simulink model "pid_handle_statico"  (R2018b)
settings: Solver=VariableStepAuto  StartTime=0.0  StopTime=10  RelTol=1e-3
values from neighbouring files (symbols this model uses):
  cond_init = [0, 150/180*pi, pi/3, -pi/2, -3*pi/4,-150/180*pi]'    [init.m]
  Legge = [Kp,Kd]    [LAUNCH_COMP_TORQUE_TRAJ.m]    (also in LAUNCH_PD.m = [Kp Kd]; LAUNCH_PD_TRAJ.m)
  param = param'    [init.m]
  q_position_f = [45/180*pi, 30*pi/180, 60*pi/180 ,90*pi/180, -45*pi/180, 330*pi/180]'    [init.m]
settings Model: Creator=Utente  LastModifiedBy=Utente

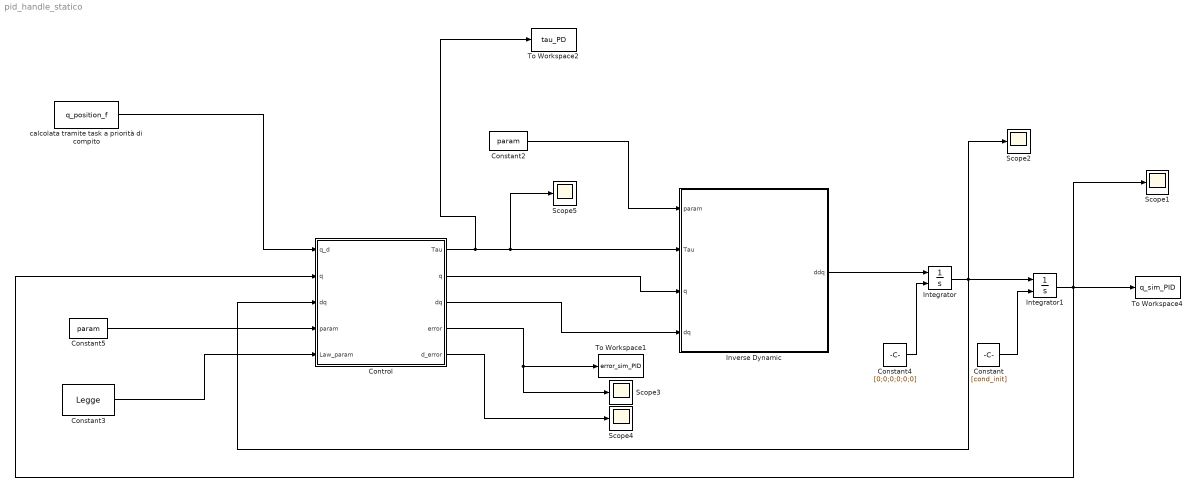
== system pid_handle_statico ==
  Constant : Constant  Value=[cond_init]
  Constant2 : Constant  Value=param
  Constant3 : Constant  Value=Legge
  Constant4 : Constant  Value=[0;0;0;0;0;0]
  Constant5 : Constant  Value=param
  Control : MATLAB Function  TreatAsAtomicUnit=on
  Integrator : Integrator  InitialConditionSource=external  InitialCondition=[0;0;0;0;0;0]
  Integrator1 : Integrator  InitialConditionSource=external
  Inverse Dynamic : MATLAB Function  TreatAsAtomicUnit=on
  Scope{1..5} (5 alike) : Scope
  To Workspace1 : ToWorkspace  VariableName=error_sim_PID  SaveFormat=Structure With Time  SampleTime=-1
      settings: Save2DSignal=2-D array (concatenate along first dimension)
  To Workspace2 : ToWorkspace  VariableName=tau_PD  SaveFormat=Structure With Time  SampleTime=-1
      settings: Save2DSignal=2-D array (concatenate along first dimension)
  To Workspace4 : ToWorkspace  VariableName=q_sim_PID  SaveFormat=Structure With Time  SampleTime=-1
      settings: Save2DSignal=2-D array (concatenate along first dimension)
  calcolata tramite task a priorità di compito : Constant  Value=q_position_f
  wires:
  Constant2/1 -> Inverse Dynamic/1(param)
  Constant3/1 -> Control/5(Law_param)
  Control/1(Tau) -> To Workspace2/1, Scope5/1, Inverse Dynamic/2(Tau)
  Control/2(q) -> Inverse Dynamic/3(q)
  Integrator/1 -> Control/3("dq "), Integrator1/1, Scope2/1
  Inverse Dynamic/1(ddq) -> Integrator/1
  Constant/1 -> Integrator1/2
  Integrator1/1 -> Control/2("q "), To Workspace4/1, Scope1/1
  Constant4/1 -> Integrator/2
  Control/3(dq) -> Inverse Dynamic/4(dq)
  calcolata tramite task a priorità di compito/1 -> Control/1(q_d)
  Constant5/1 -> Control/4(param)
  Control/4(error) -> To Workspace1/1, Scope3/1
  Control/5(d_error) -> Scope4/1

== matlab function pid_handle_statico/Control ==
  data: q_d input; q input; dq input; Tau output; param input; Law_param input; q output; dq output; error output; d_error output
function [Tau,q,dq, error, d_error] = ControlLaw(q_d, q, dq,  param, Law_param)

Kp = Law_param(1)*eye(size(q,1));
Kd = Law_param(2)*eye(size(dq,1));

[~,~,G] = Dinamica_new(param,q,dq);

error = q_d - q;
d_error = - dq;

Tau = Kp*error + G - Kd*dq;

end

== matlab function pid_handle_statico/Inverse Dynamic ==
  data: param input; Tau input; ddq output; q input; dq input
function ddq = inverseD(param,Tau,q,dq)

    [B,C,G] = Dinamica(param,q,dq);
    tot = Tau - C*dq - G;
    
    ddq = B\(tot);
    
end
